simulink model "JointSpacePD"  (R2018b)
settings: Solver=ode4  StartTime=0.0  StopTime=50  FixedStep=1e-3  RelTol=1e-3  EnableMultiTasking=on
settings Model: Creator=Asus  LastModifiedBy=batuhantoker
settings DataIOCC: LimitDataPoints=on
settings OptimizationCC: LifeSpan=inf
settings DebuggingCC: AllowSymbolicDim=off  SFUnexpectedBacktrackingDiag=warning  SFNoUnconditionalDefaultTransitionDiag=warning  SFExecutionAtInitializationDiag=none
settings ModelReferenceCC: PropagateSignalLabelsOutOfModel=off
settings SFSimCC: SimUseLocalCustomCode=off
settings RTWCC: RTWUseLocalCustomCode=off
settings CodeAppCC: StateflowObjectComments=on
settings GRTTargetCC: TargetLangStandard=C89/C90 (ANSI)
settings ConfigComp: CovMetricSettings=dw  CovHtmlReporting=on  CovSaveCumulativeToWorkspaceVar=on  CovSaveSingleToWorkspaceVar=on  CovExternalEMLEnable=off

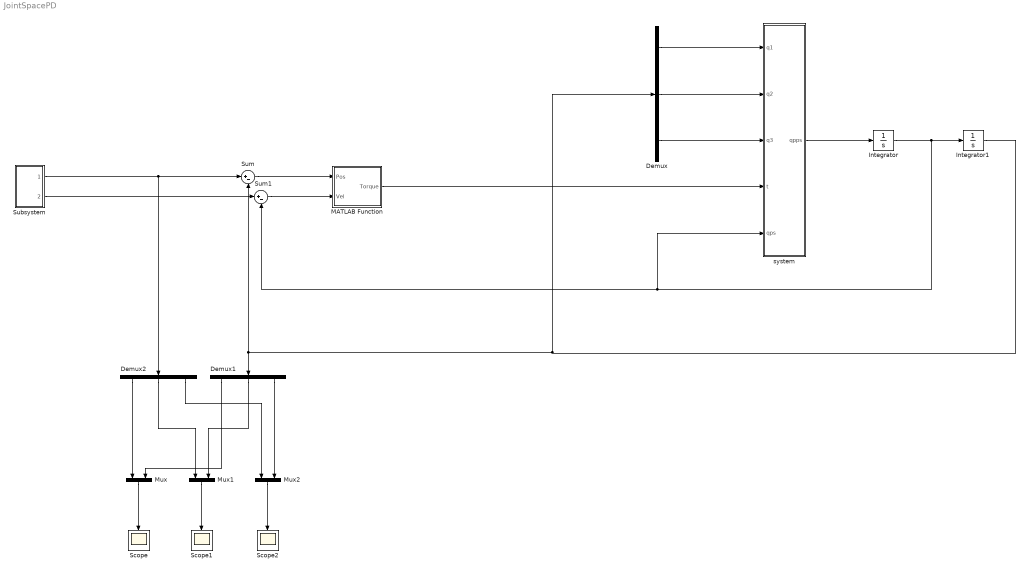
== system JointSpacePD ==
  Demux : Demux  Outputs=3
  Demux1 : Demux  Outputs=3
  Demux2 : Demux  Outputs=3
  Integrator : Integrator  InitialCondition=[0;0;0]
  Integrator1 : Integrator  InitialCondition=[0.001;0.001;0.001]
  MATLAB Function : MATLAB Function  TreatAsAtomicUnit=on
  Mux : Mux  Inputs=2
  Mux1 : Mux  Inputs=2
  Mux2 : Mux  Inputs=2
  Scope : Scope
  Scope1 : Scope
  Scope2 : Scope
  Subsystem : Subsystem
  Sum : Sum  Inputs=|+-
  Sum1 : Sum  Inputs=|+-
  system : MATLAB Function  TreatAsAtomicUnit=on
  wires:
  system/1(qpps) -> Integrator/1
  Demux/3 -> system/3(q3)
  Demux/1 -> system/1(q1)
  Demux/2 -> system/2(q2)
  Sum/1 -> MATLAB Function/1(Pos)
  Subsystem/1(Position) -> Sum/1, Demux2/1
  Sum1/1 -> MATLAB Function/2(Vel)
  Subsystem/2(Velocity) -> Sum1/1
  Demux2/1 -> Mux/1
  Mux/1 -> Scope/1
  Demux2/2 -> Mux1/1
  Demux1/2 -> Mux1/2
  Demux2/3 -> Mux2/1
  Mux2/1 -> Scope2/1
  Mux1/1 -> Scope1/1
  Demux1/1 -> Mux/2
  Integrator1/1 -> Sum/2, Demux1/1, Demux/1
  MATLAB Function/1(Torque) -> system/4(t)
  Integrator/1 -> Sum1/2, system/5(qps), Integrator1/1
  Demux1/3 -> Mux2/2

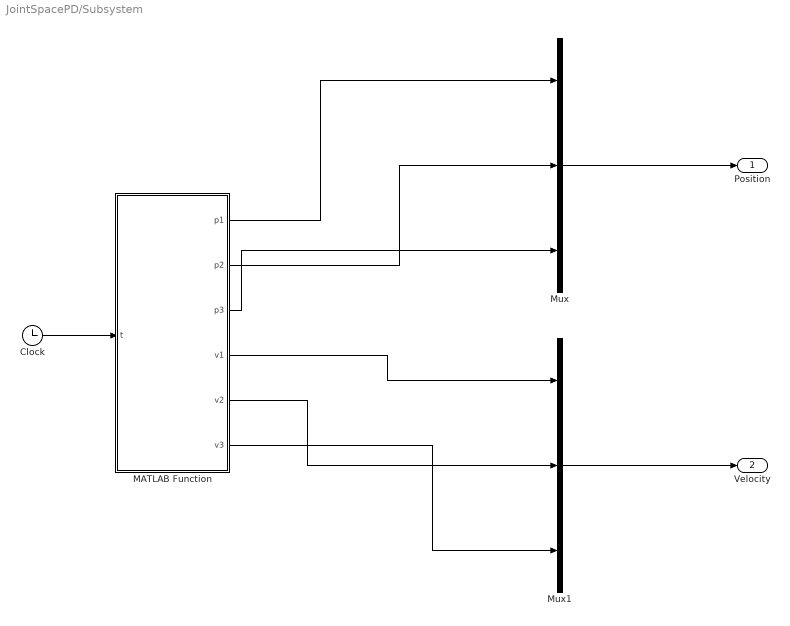
== system JointSpacePD/Subsystem ==
  Clock : Clock
  MATLAB Function : MATLAB Function  TreatAsAtomicUnit=on
  Mux : Mux  Inputs=3
  Mux1 : Mux  Inputs=3
  Position : Outport
  Velocity : Outport  Port=2
  wires:
  MATLAB Function/3(p3) -> Mux/3
  MATLAB Function/2(p2) -> Mux/2
  Mux/1 -> Position/1
  Mux1/1 -> Velocity/1
  MATLAB Function/4(v1) -> Mux1/1
  MATLAB Function/5(v2) -> Mux1/2
  MATLAB Function/6(v3) -> Mux1/3
  MATLAB Function/1(p1) -> Mux/1
  Clock/1 -> MATLAB Function/1(t)

== matlab function JointSpacePD/Subsystem/MATLAB Function ==
  data: t input; p1 output; p2 output; p3 output; v1 output; v2 output; v3 output
function [p1,p2,p3,v1,v2,v3] = Source(t)
p1 = 10*sin(0.1*t);
p2 = 10*cos(0.1*t);
p3 = 10;

v1 = cos(0.1*t);
v2 = -sin(0.1*t);
v3 = 0;

== matlab function JointSpacePD/MATLAB Function ==
  data: Pos input; Torque output; Vel input
function Torque = PD(Pos,Vel)
Kp1 = 5e6;
Kd1 = 2e6;
Torque1 = Kp1*Pos(1) + Kd1*Vel(1) ;
Kp2 = 5e6;
Kd2 = 2e6;
Torque2 = Kp2*Pos(2) + Kd2*Vel(2) ;
Kp3 = 5e6;
Kd3 = 2e6;
Torque3= Kp3*Pos(3) + Kd3*Vel(3) ;

Torque = [Torque1;Torque2;Torque3];

== matlab function JointSpacePD/system ==
  data: q1 input; q2 input; q3 input; t input; qps input; qpps output
function qpps= fcn(q1, q2, q3, t, qps)

%inertia corilois and gravity matrix terms are taken from appendix I

%masses of links
m1 = 258.22;
m2 = 57.56;
m3 = 47.17;

mA = m1;
mB = m2;
mC = m3;

%inertia matirices of the links
I1 = [290212.21, 0, 0; 0, 275331.77, 0; 0, 0, 509323.35];
I2 = [7409.27 0 0; 0 52876.31 -0.01; 0 -0.01 50680.51];
I3 = [3801.21 -0.03 -0.24; -0.03 87085.96 -0.02; -0.24 -0.02 86685.11];

IA11 = I1(1,1);
IA12 = I1(1,2);
IA13 = I1(1,3);
IA21 = I1(2,1);
IA22 = I1(2,2);
IA23 = I1(2,3);
IA31 = I1(3,1);
IA32 = I1(3,2);
IA33 = I1(3,3);

IB11 = I2(1,1);
IB12 = I2(1,2);
IB13 = I2(1,3);
IB21 = I2(2,1);
IB22 = I2(2,2);
IB23 = I2(2,3);
IB31 = I2(3,1);
IB32 = I2(3,2);
IB33 = I2(3,3);

IC11 = I3(1,1);
IC12 = I3(1,2);
IC13 = I3(1,3);
IC21 = I3(2,1);
IC22 = I3(2,2);
IC23 = I3(2,3);
IC31 = I3(3,1);
IC32 = I3(3,2);
IC33 = I3(3,3);

%inertia matrix
m11 = IA33 + IB33 + IC33 + 2437.6881917025 * mB  ...
    + 4917.62782564 * mC * (cos(q2 + q3)^2 + 1.982816331884774 * cos(q2)^2 ...
    + 2.816250224596368 * cos(q2) * cos(q2 + q3)) + sin(q2 + q3) * (IC11 * sin(q2 + q3) ...
    + 2 * IC31 * cos(q2 + q3) - IC33 - sin(q2 + q3)) + sin(q2) - (IB11 - sin(q2) ...
    + 2 * IB31 * cos(q2) - 2437.6881917025 * mB * sin(q2) - IB33 * sin(q2));

m12 = -IB12 * sin(q2) - IB23 * cos(q2) - IC12 * sin(q2 + q3) - IC23 * cos(q2 + q3);
m13 = -IC12 * sin(q2 + q3) - IC23 * cos(q2 + q3);
m21 = -IB12 * sin(q2) - IB23 * cos(q2) - IC12 * sin(q2 + q3) - IC23 * cos(q2 + q3);
m22 = IB22 + IC22 + 2437.6881917025 * mB + 13849.27046844 * mC * (1.059144640569812 + cos(q3));
m23 = IC22 + 4917.62782564 * mC * (1 + 1.408125112298184 * cos(q3));
m31 = -IC12 * sin(q2 + q3) - IC23 * cos(q2 + q3);
m32 = IC22 + 4917.62782564 * mC * (1 + 1.408125112298184 * cos(q3));
m33 = IC22 + 4917.62782564 * mC;

M = [m11, m12, m13; m21, m22, m23; m31, m32, m33];

%coriolis matrix 
c11 = cos(q2)*(IB31*cos(q2)-2437.6881917025*mB*sin(q2))+2*sin(q2+q3)*(IC11*cos(q2+q3)-IC31*sin(q2+q3))...
    +2*cos(q2+q3)*(IC31*cos(q2+q3)-IC33*sin(q2+q3))+sin(q2)*(IB11*cos(q2)-IB31*sin(q2)-IB33*cos(q2))...
    -6924.635234220001*mC*(sin(q3+ 2 * q2) + 1.408125112298184 * sin(q2) * cos(q2)) ...
    - 6924.635234220001 * mC * sin(q2 + q3) * (cos(q2) + 1.420328337682881 * cos(q2 + q3));

c12 = IB23 * sin(q2) + 2 * IC23 * sin(q2 + q3) + cos(q2) * (IB31 * cos(q2)... 
    - 2437.6881917025 * mB * sin(q2)) + sin(q2 + q3) * (IC11 * cos(q2 + q3) - IC31 * sin(q2 + q3)) ...
    + cos(q2 + q3) * (IC31 * cos(q2 + q3) - IC33 * sin(q2 + q3))...
    + sin(q2) * (IB11 * cos(q2) - IB31 * sin(q2) - IB33 * cos(q2)) ...
    - IB12 * cos(q2) - 2 * IC12 * cos(q2 + q3) ...
    - 4917.62782564 * mC * (1.408125112298184 * sin(q3 + 2 * q2) ...
    + 1.982816331884774 * sin(q2) * cos(q2) + sin(q2 + q3) * cos(q2 + q3));

c13 = 2 * IC23 * sin(q2 + q3) + sin(q2 + q3) * (IC11 * cos(q2 + q3) - IC31 * sin(q2 + q3)) ...
    + cos(q2 + q3) * (IC31 * cos(q2 + q3) - IC33 * sin(q2 + q3)) - 2 * IC12 * cos(q2 + q3) ...
    - 4917.62782564 * mC * sin(q2 + q3) * (cos(q2 + q3) + 1.408125112298184 * cos(q2));

c21 = 4917.62782564 * mC * (1.408125112298184 * sin(q3 + 2 * q2) ...
    + 1.982816331884774 * sin(q2) * cos(q2) + sin(q2 + q3) * cos(q2 + q3)) ...
    - cos(q2) * (IB31 * cos(q2) - 2437.6881917025 * mB * sin(q2)) ...
    - sin(q2 + q3) * (IC11 * cos(q2 + q3) - IC31 * sin(q2 + q3)) ...
    -cos(q2 + q3) * (IC31 * cos(q2 + q3) - IC33 * sin(q2 + q3)) ...
    - sin(q2) * (IB11 * cos(q2) - IB31 * sin(q2) - IB33 * cos(q2));

c22 = -6924.63523422 * mC * sin(q3);

c23 = -13849.27046844 * mC * sin(q3);

c31 = 4917.62782564 * mC * sin(q2 + q3) * (cos(q2 + q3) + 1.408125112298184 * cos(q2))...
    - sin(q2 + q3) * (IC11 * cos(q2 + q3) - IC31 * sin(q2 + q3)) ...
    - cos(q2 + q3) * (IC31 * cos(q2 + q3) - IC33 * sin(q2 + q3));

c32 = 6924.63523422 * mC * sin(q3);

c33 = 0;

C = [c11, c12, c13; c21, c22, c23; c31, c32, c33];

%gravity matrix
g = 9810;

g1 = 0;
g2 = 49.37295 * g * (mB + 2 * mC) * cos(q2);
g3 = 70.1258 * g * mC * cos(q3);


Cqp = C * qps;
%G = [g1; g2; g3];

qpps = inv(M)*(t - Cqp)% - %G)
